simulink model "Arduino"  (R2023b)
settings: Solver=VariableStepAuto  StartTime=0.0  StopTime=150  RelTol=1e-3
settings Model: Creator=user  LastModifiedBy=user

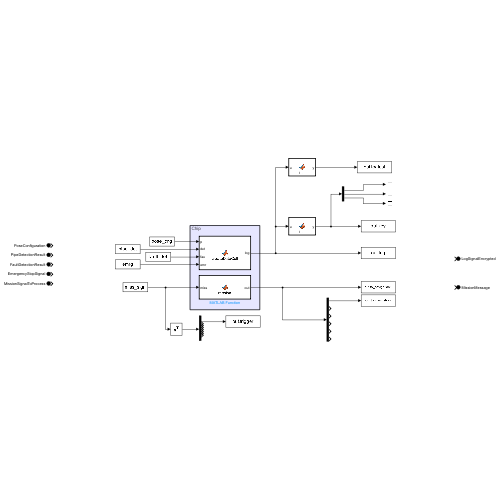
[thumbnail: Simulink's stored preview of the top-level diagram]
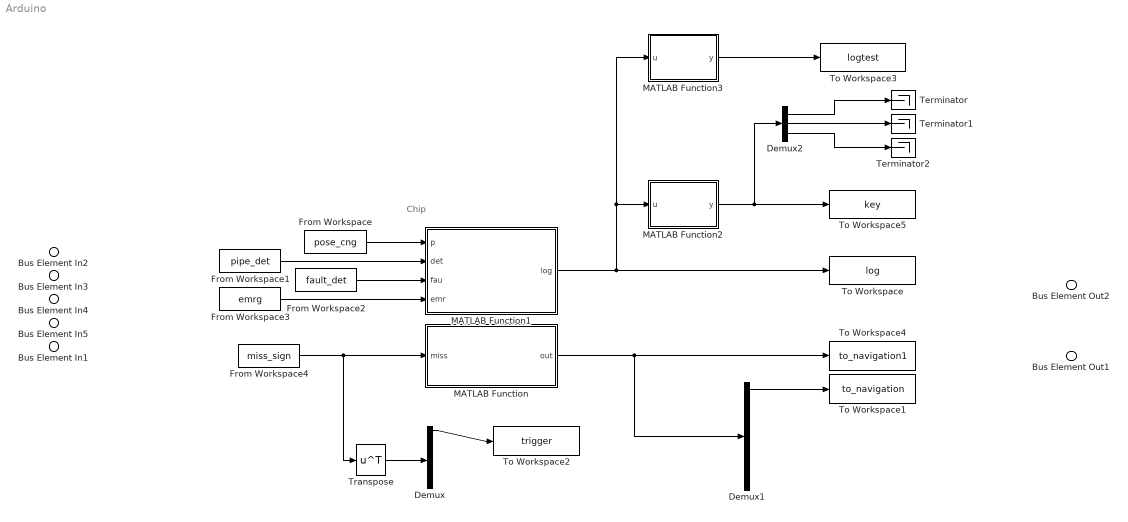
== system Arduino ==
  note: Chip
  Bus Element In2 : Inport  PortName=PoseConfiguration
  Bus Element In3 : Inport  Port=2  PortName=PipeDetectionResult
  Bus Element In4 : Inport  Port=3  PortName=FaultDetectionResult
  Bus Element In5 : Inport  Port=4  PortName=EmergencyStopSignal
  Bus Element In1 : Inport  Port=5  PortName=MissionSignalToProcess
  Demux : Demux  Outputs=8
  Demux1 : Demux  Outputs=6
  Demux2 : Demux  Outputs=3
  From Workspace : FromWorkspace  VariableName=pose_cng  SampleTime=1
  From Workspace1 : FromWorkspace  VariableName=pipe_det  SampleTime=1
  From Workspace2 : FromWorkspace  VariableName=fault_det  SampleTime=1
  From Workspace3 : FromWorkspace  VariableName=emrg  SampleTime=1
  From Workspace4 : FromWorkspace  VariableName=miss_sign  SampleTime=1
  MATLAB Function : MATLAB Function  TreatAsAtomicUnit=on
  MATLAB Function1 : MATLAB Function  TreatAsAtomicUnit=on
  MATLAB Function2 : MATLAB Function  TreatAsAtomicUnit=on
  MATLAB Function3 : MATLAB Function  TreatAsAtomicUnit=on
  Terminator : Terminator
  Terminator1 : Terminator
  Terminator2 : Terminator
  To Workspace : ToWorkspace  VariableName=log  SaveFormat=Timeseries  SampleTime=1
  To Workspace1 : ToWorkspace  VariableName=to_navigation  SaveFormat=Timeseries  SampleTime=1
  To Workspace2 : ToWorkspace  VariableName=trigger  SaveFormat=Timeseries  SampleTime=-1
  To Workspace3 : ToWorkspace  VariableName=logtest  SaveFormat=Timeseries  SampleTime=1
  To Workspace4 : ToWorkspace  VariableName=to_navigation1  SaveFormat=Timeseries  SampleTime=1
  To Workspace5 : ToWorkspace  VariableName=key  SaveFormat=Timeseries  SampleTime=1
  Transpose : Math  Operator=transpose
  Bus Element Out2 : Outport  PortName=LogSignalEncrypted
  Bus Element Out1 : Outport  Port=2  PortName=MissionMessage
  wires:
  From Workspace3/1 -> MATLAB Function1/4(emr)
  From Workspace1/1 -> MATLAB Function1/2(det)
  From Workspace/1 -> MATLAB Function1/1(p)
  From Workspace2/1 -> MATLAB Function1/3(fau)
  From Workspace4/1 -> Transpose/1, MATLAB Function/1(miss)
  MATLAB Function1/1(log) -> MATLAB Function3/1(u), MATLAB Function2/1(u), To Workspace/1
  Transpose/1 -> Demux/1
  Demux/1 -> To Workspace2/1
  MATLAB Function/1(out) -> Demux1/1, To Workspace4/1
  Demux1/1 -> To Workspace1/1
  MATLAB Function2/1(y) -> Demux2/1, To Workspace5/1
  Demux2/1 -> Terminator/1
  Demux2/2 -> Terminator1/1
  Demux2/3 -> Terminator2/1
  MATLAB Function3/1(y) -> To Workspace3/1

== matlab function Arduino/MATLAB Function1 ==
  data: p input; log output; det input; fau input; emr input
function log = createDataCell(p, det, fau, emr)

   y = [12, 34, 1234; p(1,1), p(2,1), p(3,1); det, fau, emr];


log = y;

== matlab function Arduino/MATLAB Function ==
  data: miss input; out output
function out = mission(miss)
  out = zeros(1, 6);
  if miss(1) == 1
      if miss(2) == 1234
          out(1:6) = [miss(3:5) miss(6:8)];
      else
          out(1:6) = [-100 -100 -100 -100 -100 -100];
      end
  else
      out = [-1 -1 -1 -1 -1 -1];
  end
end

== matlab function Arduino/MATLAB Function2 ==
  data: u input; y output
function y = fcn(u)
   row = u(1,:);
y = row;

== matlab function Arduino/MATLAB Function3 ==
  data: u input; y output
function y = fcn(u)
   dims = size(u);
   num_element = dims(1)*dims(2);
y = num_element;
